simulink model "Kff"  (R2024b)
settings: Solver=VariableStepAuto  StartTime=0.0  StopTime=10.0  RelTol=1e-3
settings Model: Creator=Ilya  LastModifiedBy=Ilya

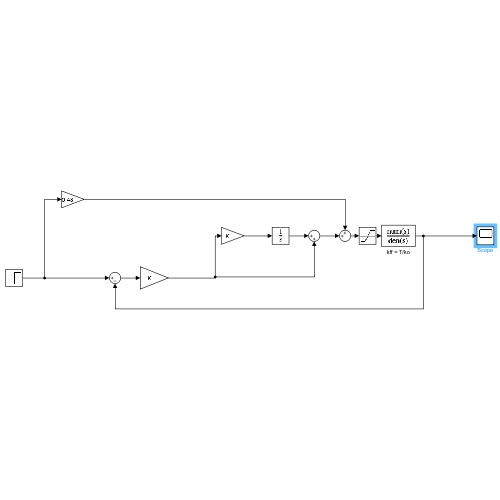
[thumbnail: Simulink's stored preview of the top-level diagram]
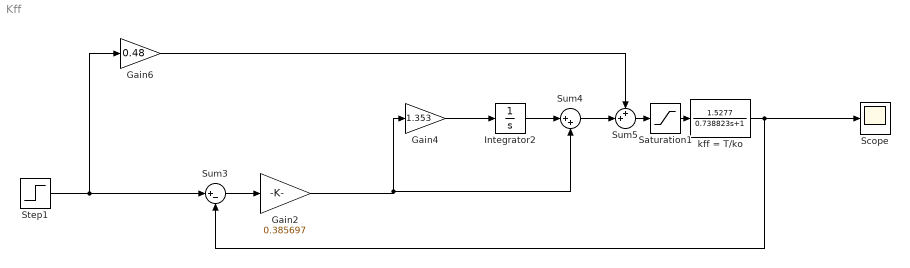
== system Kff ==
  Gain2 : Gain  Gain=0.385697
  Gain4 : Gain  Gain=1.353
  Gain6 : Gain  Gain=0.48
  Integrator2 : Integrator
  Saturation1 : Saturate  UpperLimit=1000  LowerLimit=0
  Scope : Scope
  Step1 : Step  Time=0  After=100  SampleTime=0
  Sum3 : Sum  Inputs=|+-
  Sum4 : Sum  Inputs=|++
  Sum5 : Sum  Inputs=++|
  kff = T/ko : TransferFcn  Numerator=[1.5277]  Denominator=[0.738823 1]
  wires:
  Sum5/1 -> Saturation1/1
  Sum4/1 -> Sum5/2
  Sum3/1 -> Gain2/1
  Saturation1/1 -> kff = T/ko/1
  Integrator2/1 -> Sum4/1
  Gain4/1 -> Integrator2/1
  Gain6/1 -> Sum5/1
  Gain2/1 -> Gain4/1, Sum4/2
  kff = T/ko/1 -> Scope/1, Sum3/2
  Step1/1 -> Gain6/1, Sum3/1
